simulink model "smdfk"  (R2016a)
settings: Solver=FixedStepDiscrete  StartTime=0.0  StopTime=10.0  FixedStep=0.1  RelTol=1e-3
settings Model: Creator=Samvrit  LastModifiedBy=Samvrit
settings SolverCC: AutoInsertRateTranBlk=on
settings DataIOCC: LimitDataPoints=on
settings DebuggingCC: AllowSymbolicDim=off
settings ConfigComp: CovModelRefEnable=Off  CovSFcnEnable=off

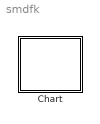
== system smdfk ==
  Chart : Stateflow chart  TreatAsAtomicUnit=on

== stateflow chart smdfk/Chart ==
  state IDLE
  state SIMULATE_ROBOT
    entry: using joint angles
  state CALCULATE_TRANSFORMATION_MATRIX
    entry: using joint angles j1, j2, j3
  state CALCULATE_TAIT_BRYAN_ANGLES
    entry: using transformation matrix
  (default) -> IDLE
  IDLE -> CALCULATE_TRANSFORMATION_MATRIX [order 1] : createrotmatrix_button_press
  CALCULATE_TRANSFORMATION_MATRIX -> IDLE : transformation_matrix_creation
  IDLE -> CALCULATE_TAIT_BRYAN_ANGLES [order 2] : compute_button_press
  CALCULATE_TAIT_BRYAN_ANGLES -> IDLE : tait_bryan_angles_calculation
  IDLE -> SIMULATE_ROBOT [order 3] : simulate_button_press
  SIMULATE_ROBOT -> IDLE : simulation_completion
